simulink model "model_4_lqg"  (R2021b)
settings: Solver=VariableStepAuto  StartTime=0.0  StopTime=10  RelTol=1e-3
values from neighbouring files (symbols this model uses):
  A = [-6, -25, -35, -10; 0, -9, -15, 0; 0, 6, 9, 0; 4, 17, 26, 6]    [task_1.m]    (also in task_2.m; task_3.m; task_4.m)
  B = [16, 0; 3, 0; -3, 0; -11, 0]    [task_1.m]    (also in task_2.m; task_3.m = [0; 0; 0; 0]; task_4.m)
  C = eye(4)    [task_1.m]    (also in task_2.m; task_3.m = [2, 2, 0, 4; 0, 3, 6, 0]; task_4.m = [2, 2, 0, 4; 0, 3, 6, 0])
  D = zeros(4, 2)    [task_1.m]    (also in task_2.m; task_3.m = zeros(2, 1); task_4.m = [0, 0; 0, 4])
  K = -inv(R_1)*B'*P_1    [task_4.m]
  L = -P*C'*inv(R)    [task_3.m]    (also in task_4.m)
  x0 = [1000; -1000; 1000; -1000]    [task_1.m]    (also in task_2.m; task_3.m = [10; -10; 5; -5]; task_4.m = [10; -10; 5; -5])
  x_0 = [5; 10; -5; 10]    [task_3.m]    (also in task_4.m)
settings Model: Creator=vital  LastModifiedBy=vital

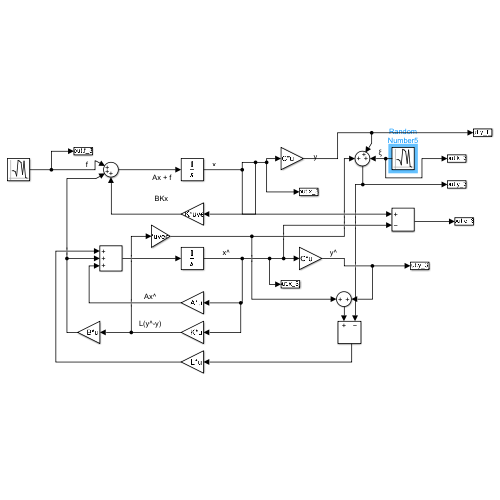
[thumbnail: Simulink's stored preview of the top-level diagram]
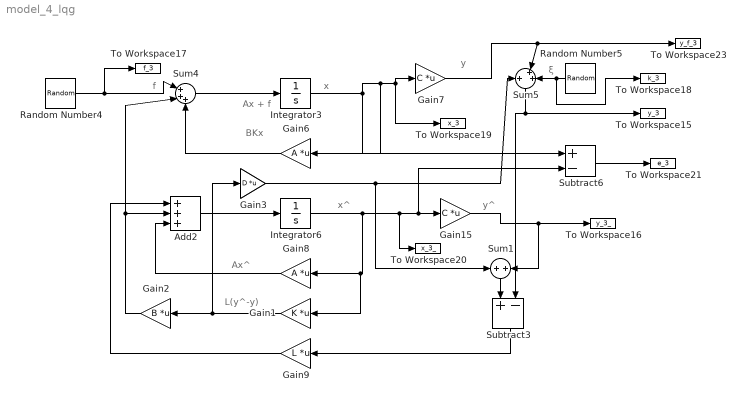
== system model_4_lqg ==
  note: Ax^
  note: BKx
  note: x^
  note: L(y^-y)
  note: x
  note: f
  note: y^
  note: Ax + f
  note: y
  note: ξ
  Add2 : Sum  Inputs=+++
  Gain1 : Gain  Gain=K  Multiplication=Matrix(K*u)
  Gain15 : Gain  Gain=C  Multiplication=Matrix(K*u)
  Gain2 : Gain  Gain=B  Multiplication=Matrix(K*u)
  Gain3 : Gain  Gain=D  Multiplication=Matrix(K*u) (u vector)
  Gain6 : Gain  Gain=A  Multiplication=Matrix(K*u) (u vector)
  Gain7 : Gain  Gain=C  Multiplication=Matrix(K*u)
  Gain8 : Gain  Gain=A  Multiplication=Matrix(K*u)
  Gain9 : Gain  Gain=L  Multiplication=Matrix(K*u)
  Integrator3 : Integrator  InitialCondition=x0
  Integrator6 : Integrator  InitialCondition=x_0
  Random Number4 : RandomNumber  Variance=5  Seed=[13; 14; 15; 16]  SampleTime=0000.1
  Random Number5 : RandomNumber  Variance=25  Seed=[17; 18]  SampleTime=0000.1
  Subtract3 : Sum  Inputs=+-
  Subtract6 : Sum  Inputs=+-
  Sum1 : Sum  Inputs=+|+
  Sum4 : Sum  Inputs=|+++
  Sum5 : Sum  Inputs=+|++
  To Workspace15 : ToWorkspace  VariableName=y_3  SaveFormat=Timeseries  SampleTime=-1
  To Workspace16 : ToWorkspace  VariableName=y_3_  SaveFormat=Timeseries  SampleTime=-1
  To Workspace17 : ToWorkspace  VariableName=f_3  SaveFormat=Timeseries  SampleTime=-1
  To Workspace18 : ToWorkspace  VariableName=k_3  SaveFormat=Timeseries  SampleTime=-1
  To Workspace19 : ToWorkspace  VariableName=x_3  SaveFormat=Timeseries  SampleTime=0.0001
  To Workspace20 : ToWorkspace  VariableName=x_3_  SaveFormat=Timeseries  SampleTime=-1
  To Workspace21 : ToWorkspace  VariableName=e_3  SaveFormat=Timeseries  SampleTime=-1
  To Workspace23 : ToWorkspace  VariableName=y_f_3  SaveFormat=Timeseries  SampleTime=-1
  wires:
  Gain7/1 -> Sum5/2, To Workspace23/1
  Sum4/1 -> Integrator3/1
  Add2/1 -> Integrator6/1
  Gain15/1 -> Sum1/2, To Workspace16/1
  Random Number4/1 -> Sum4/1, To Workspace17/1
  Sum5/1 -> To Workspace15/1, Subtract3/2
  Integrator3/1 -> To Workspace19/1, Gain7/1, Gain6/1, Subtract6/1
  Random Number5/1 -> Sum5/3, To Workspace18/1
  Integrator6/1 -> Gain1/1, Gain8/1, To Workspace20/1, Subtract6/2, Gain15/1
  Subtract6/1 -> To Workspace21/1
  Subtract3/1 -> Gain9/1
  Gain6/1 -> Sum4/3
  Gain8/1 -> Add2/3
  Gain9/1 -> Add2/1
  Gain1/1 -> Gain3/1, Gain2/1
  Gain2/1 -> Sum4/2, Add2/2
  Gain3/1 -> Sum1/1, Sum5/1
  Sum1/1 -> Subtract3/1
